simulink model "rpmTest"  (R2015b)
settings: Solver=FixedStepDiscrete  StartTime=0.0  StopTime=Inf  RelTol=1e-3
libraries: frdmkl25zlib x3
settings Model: ExtModeTrigDuration=5  Creator=dc315  LastModifiedBy=dc315
settings OptimizationCC: OptimizeModelRefInitCode=on  LifeSpan=1  MaxStackSize=64
settings HardwareCC: ProdBitPerPointer=32  ProdLargestAtomicInteger=Long  ProdLargestAtomicFloat=Double  ProdWordSize=32  ProdHWDeviceType=ARM Compatible->ARM Cortex
settings RTWCC: SystemTargetFile=ert.tlc  TemplateMakefile=ert_default_tmf  Description=Embedded Coder  Toolchain=GNU Tools for ARM Embedded Processors
settings CodeAppCC: IgnoreCustomStorageClasses=off
settings ERTTargetCC: GenerateSampleERTMain=on

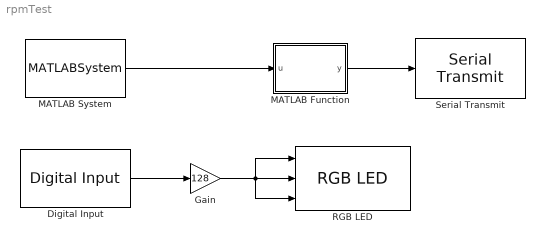
== system rpmTest ==
  Digital Input : frdmkl25zlib/Digital Input  WhichPin=D4  SampleTime=0.1
  Gain : Gain  Gain=128
  MATLAB Function : MATLAB Function  TreatAsAtomicUnit=on
  MATLAB System : MATLABSystem  System=freedomboard.rpmSensor  SimulateUsing=Code generation
      mask Type: freedomboard.rpmSensor
      mask Display:
      | disp('rpmSensor');
      | port_label('output',1,'rpm');
  RGB LED : frdmkl25zlib/RGB LED
  Serial Transmit : frdmkl25zlib/Serial Transmit  uart=UART0  sendmode=putc
  wires:
  MATLAB Function/1(y) -> Serial Transmit/1
  MATLAB System/1 -> MATLAB Function/1(u)
  Digital Input/1 -> Gain/1
  Gain/1 -> RGB LED/3, RGB LED/1, RGB LED/2

== matlab function rpmTest/MATLAB Function ==
  data: u input; y output
function y = fcn(u)
%#codegen

y = typecast(u,'uint8');
